simulink library "Banshee_SEL751_Woodward_lib"  (Simulink 8.1)
settings: Solver=ode45  StartTime=0.0  StopTime=10.0  RelTol=1e-3
undefined symbols (not defined in the file): fdesignblkfcn, gcbh
libraries: rtio_opalrt_common x13, simulink x13, rtio_opalrt_op5142ex1 x12, simulink_extras x8, dspswit3 x6
(part 1 of 2)
settings Model: Creator=re25624  LastModifiedBy=re25624

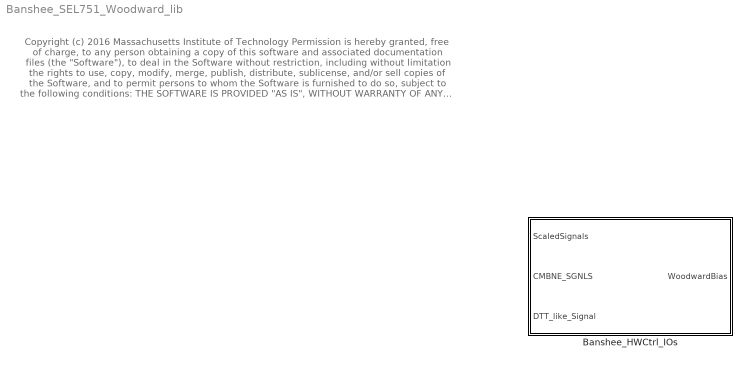
== system Banshee_SEL751_Woodward_lib ==
  note: Copyright (c) 2016 Massachusetts Institute of Technology
      | Permission is hereby granted, free of charge, to any person obtaining a copy of this software and associated documentation files (the "Software"), to deal
      | in the Software without restriction, including without limitation the rights to use, copy, modify, merge, publish, distribute, sublicense, and/or sell copies of the
      | Software, and to permit persons to whom the Software is furnished to do so, subject to the following conditions:
      |
      | THE SOFTWARE IS PROVIDED "AS IS", WITHOUT WARRANTY OF ANY KIND, EXPRESS OR IMPLIED, INCLUDING BUT NOT LIMITED TO THE
      | WARRANTIES OF MERCHANTABILITY, FITNESS FOR A PARTICULAR PURPOSE AND NONINFRINGEMENT. IN NO EVENT SHALL THE AUTHORS
      | OR COPYRIGHT HOLDERS BE LIABLE FOR ANY CLAIM, DAMAGES OR OTHER LIABILITY, WHETHER IN AN ACTION OF CONTRACT, TORT OR
      | OTHERWISE, ARISING FROM, OUT OF OR IN CONNECTION WITH THE SOFTWARE OR THE USE OR OTHER DEALINGS IN THE SOFTWARE
  Banshee_HWCtrl_IOs : Subsystem

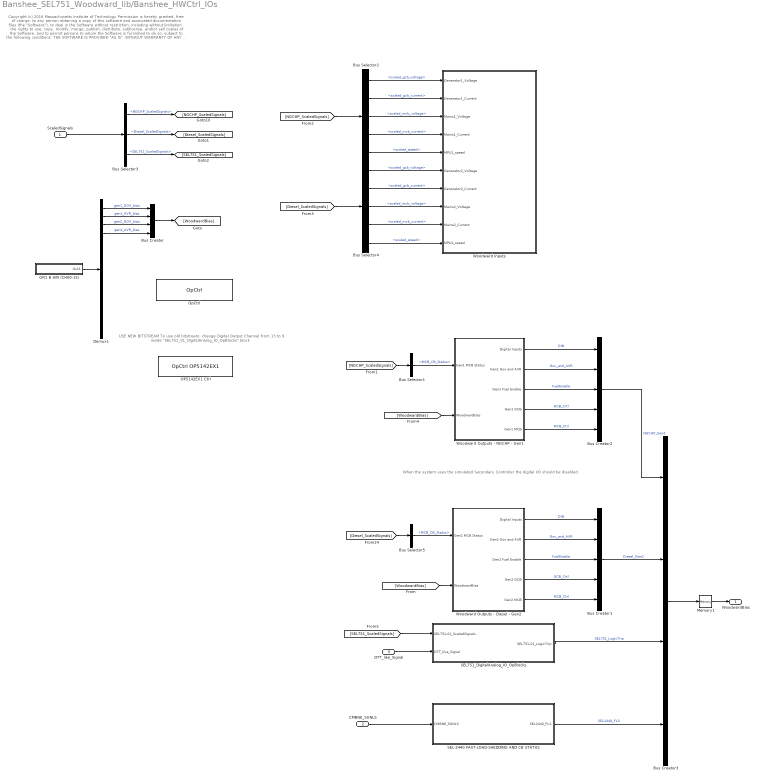
== system Banshee_SEL751_Woodward_lib/Banshee_HWCtrl_IOs ==
  note: USE NEW  BITSTREAM
      | To use old bitstream, change Digital Output Channel from 13 to 9 inside
      | "SEL751_01_DigitalAnalog_IO_OpBlocks" block
  note: Copyright (c) 2016 Massachusetts Institute of Technology
      | Permission is hereby granted, free of charge, to any person obtaining a copy of this software and associated documentation files (the "Software"), to deal
      | in the Software without restriction, including without limitation the rights to use, copy, modify, merge, publish, distribute, sublicense, and/or sell copies of the
      | Software, and to permit persons to whom the Software is furnished to do so, subject to the following conditions:
      |
      | THE SOFTWARE IS PROVIDED "AS IS", WITHOUT WARRANTY OF ANY KIND, EXPRESS OR IMPLIED, INCLUDING BUT NOT LIMITED TO THE
      | WARRANTIES OF MERCHANTABILITY, FITNESS FOR A PARTICULAR PURPOSE AND NONINFRINGEMENT. IN NO EVENT SHALL THE AUTHORS
      | OR COPYRIGHT HOLDERS BE LIABLE FOR ANY CLAIM, DAMAGES OR OTHER LIABILITY, WHETHER IN AN ACTION OF CONTRACT, TORT OR
      | OTHERWISE, ARISING FROM, OUT OF OR IN CONNECTION WITH THE SOFTWARE OR THE USE OR OTHER DEALINGS IN THE SOFTWARE
  note: When the system uses the simulated
      | Secondary Controller the digital I/O
      | should be disabled.
  ScaledSignals : Inport
  CMBNE_SGNLS : Inport  Port=2
  DTT_like_Signal : Inport  Port=3
  Bus Creator : BusCreator
  Bus Creator1 : BusCreator  Inputs=5
  Bus Creator2 : BusCreator  Inputs=5
  Bus Creator3 : BusCreator
  Bus Selector1 : BusSelector  OutputSignals=MCB_CB_Status
  Bus Selector2 : BusSelector  OutputSignals=scaled_gcb_voltage,scaled_gcb_current,scaled_mcb_voltage,scaled_mcb_current,scaled_speed
  Bus Selector3 : BusSelector  OutputSignals=NGCHP_ScaledSignals,Diesel_ScaledSignals,SEL751_ScaledSignals
  Bus Selector4 : BusSelector  OutputSignals=scaled_gcb_voltage,scaled_gcb_current,scaled_mcb_voltage,scaled_mcb_current,scaled_speed
  Bus Selector5 : BusSelector  OutputSignals=MCB_CB_Status
  Demux1 : Demux  Outputs=16
  GR1 B AIN (CH00-15) : Subsystem
  Memory1 : Memory
  OP5142EX1 Ctrl : rtio_opalrt_op5142ex1/OpCtrl OP5142EX1  CtrlName='OP5142EX1 Ctrl'  boardid=1  BitstreamFilename=OP5142_1-EX-0000-2_3_4_54-16AIO_48AO_32DO_16DIO_16selDIO_CD-FF-01.bin  numconfig=-1  mode=Slave  externalClock=off  decimRtsi=0  calibIO=off  SampleTime=0  loadinport=-1
  OpCtrl : rtio_opalrt_common/OpCtrl  CtrlName='OpCtrl'  boardid=0  BitstreamFilename=VC707_2-EX-0001-2_3_2_20-48AIO16DIO16DIOSel-02-01.bin  numconfig=-1  mode=Master  externalClock=off  decimRtsi=0  calibIO=off  SampleTime=0  loadinport=-1  BoardType=VC707  SecondaryPresent=off  sync_type=Audio
  SEL-2440 FAST-LOAD-SHEDDING AND CB STATUS : Subsystem
  SEL751_DigitalAnalog_IO_OpBlocks : Subsystem
  Woodward Inputs : Subsystem
  Woodward Outputs - Diesel - Gen2 : Subsystem
  Woodward Outputs - NGCHP - Gen1 : Subsystem
  WoodwardBias : Outport
  wires:
  DTT_like_Signal/1 -> SEL751_DigitalAnalog_IO_OpBlocks/2(DTT_like_Signal)
  SEL-2440 FAST-LOAD-SHEDDING AND CB STATUS/1(SEL2440_FLS) -> Bus Creator3/4  "SEL2440_FLS"
  CMBNE_SGNLS/1 -> SEL-2440 FAST-LOAD-SHEDDING AND CB STATUS/1(CMBNE_SGNLS)
  [SEL751_ScaledSignals] -> SEL751_DigitalAnalog_IO_OpBlocks/1(SEL751-01_ScaledSignals)
  Bus Selector3/3 -> [SEL751_ScaledSignals]  "<SEL751_ScaledSignals>"
  SEL751_DigitalAnalog_IO_OpBlocks/1(SEL751-01_LogicTrip) -> Bus Creator3/3  "SEL751_LogicTrip"
  ScaledSignals/1 -> Bus Selector3/1
  Bus Selector3/1 -> [NGCHP_ScaledSignals]  "<NGCHP_ScaledSignals>"
  Bus Selector3/2 -> [Diesel_ScaledSignals]  "<Diesel_ScaledSignals>"
  [NGCHP_ScaledSignals] -> Bus Selector2/1
  Bus Selector2/5 -> Woodward Inputs/5(MPU1_speed)  "<scaled_speed>"
  Bus Selector2/4 -> Woodward Inputs/4(Mains1_Current)  "<scaled_mcb_current>"
  Bus Selector2/3 -> Woodward Inputs/3(Mains1_Voltage)  "<scaled_mcb_voltage>"
  Bus Selector2/2 -> Woodward Inputs/2(Generator1_Current)  "<scaled_gcb_current>"
  Bus Selector2/1 -> Woodward Inputs/1(Generator1_Voltage)  "<scaled_gcb_voltage>"
  [Diesel_ScaledSignals] -> Bus Selector4/1
  Bus Selector4/1 -> Woodward Inputs/6(Generator2_Voltage)  "<scaled_gcb_voltage>"
  Bus Selector4/2 -> Woodward Inputs/7(Generator2_Current)  "<scaled_gcb_current>"
  Bus Selector4/3 -> Woodward Inputs/8(Mains2_Voltage)  "<scaled_mcb_voltage>"
  Bus Selector4/4 -> Woodward Inputs/9(Mains2_Current)  "<scaled_mcb_current>"
  Bus Selector4/5 -> Woodward Inputs/10(MPU2_speed)  "<scaled_speed>"
  GR1 B AIN (CH00-15)/1(Out1) -> Demux1/1
  Demux1/1 -> Bus Creator/1  "gen1_GOV_bias"
  Demux1/2 -> Bus Creator/2  "gen1_AVR_bias"
  Demux1/3 -> Bus Creator/3  "gen2_GOV_bias"
  Demux1/4 -> Bus Creator/4  "gen2_AVR_bias"
  Bus Selector5/1 -> Woodward Outputs - Diesel - Gen2/1(Gen2 MCB Status)  "<MCB_CB_Status>"
  [WoodwardBias] -> Woodward Outputs - Diesel - Gen2/2(WoodwardBias)
  [Diesel_ScaledSignals] -> Bus Selector5/1
  Woodward Outputs - Diesel - Gen2/2(Gen2 Gov and AVR) -> Bus Creator1/2  "Gov_and_AVR"
  Woodward Outputs - Diesel - Gen2/3(Gen2 Fuel Enable) -> Bus Creator1/3  "FuelEnable"
  Woodward Outputs - Diesel - Gen2/4(Gen2 GCB) -> Bus Creator1/4  "GCB_Crtl"
  Woodward Outputs - Diesel - Gen2/5(Gen2 MCB) -> Bus Creator1/5  "MCB_Ctrl"
  Bus Creator1/1 -> Bus Creator3/2  "Diesel_Gen2"
  Bus Creator3/1 -> Memory1/1
  Bus Creator2/1 -> Bus Creator3/1  "NGCHP_Gen1"
  Woodward Outputs - NGCHP - Gen1/1(Digital Inputs) -> Bus Creator2/1  "DIN"
  Woodward Outputs - NGCHP - Gen1/2(Gen1 Gov and AVR) -> Bus Creator2/2  "Gov_and_AVR"
  Woodward Outputs - NGCHP - Gen1/3(Gen1 Fuel Enable) -> Bus Creator2/3  "FuelEnable"
  Woodward Outputs - NGCHP - Gen1/4(Gen1 GCB) -> Bus Creator2/4  "GCB_Crtl"
  Woodward Outputs - Diesel - Gen2/1(Digital Inputs) -> Bus Creator1/1  "DIN"
  Woodward Outputs - NGCHP - Gen1/5(Gen1 MCB) -> Bus Creator2/5  "MCB_Ctrl"
  [WoodwardBias] -> Woodward Outputs - NGCHP - Gen1/2(WoodwardBias)
  [NGCHP_ScaledSignals] -> Bus Selector1/1
  Bus Selector1/1 -> Woodward Outputs - NGCHP - Gen1/1(Gen1 MCB Status)  "<MCB_CB_Status>"
  Memory1/1 -> WoodwardBias/1
  Bus Creator/1 -> [WoodwardBias]

== system Banshee_SEL751_Woodward_lib/Banshee_HWCtrl_IOs/GR1 B AIN (CH00-15) ==
  AnalogIn : rtio_opalrt_common/AnalogIn  CtrlName='OpCtrl'  portNb=1  FcnNos=Slot 1 Module B Subsection 1  size=16  maxcount=8  count=8  numchan=8  sampleTime=0
      settings: AttributesFormatString=%<CtrlName>
  AnalogIn1 : rtio_opalrt_common/AnalogIn  CtrlName='OpCtrl'  portNb=2  FcnNos=Slot 1 Module B Subsection 2  size=16  maxcount=8  count=8  numchan=8  sampleTime=0
      settings: AttributesFormatString=%<CtrlName>
  Mux6 : Mux  Inputs=2
  Terminator2 : Terminator
  Terminator3 : Terminator
  Out1 : Outport
  wires:
  AnalogIn/1 -> Mux6/1
  AnalogIn1/1 -> Mux6/2
  AnalogIn/2 -> Terminator2/1
  AnalogIn1/2 -> Terminator3/1
  Mux6/1 -> Out1/1

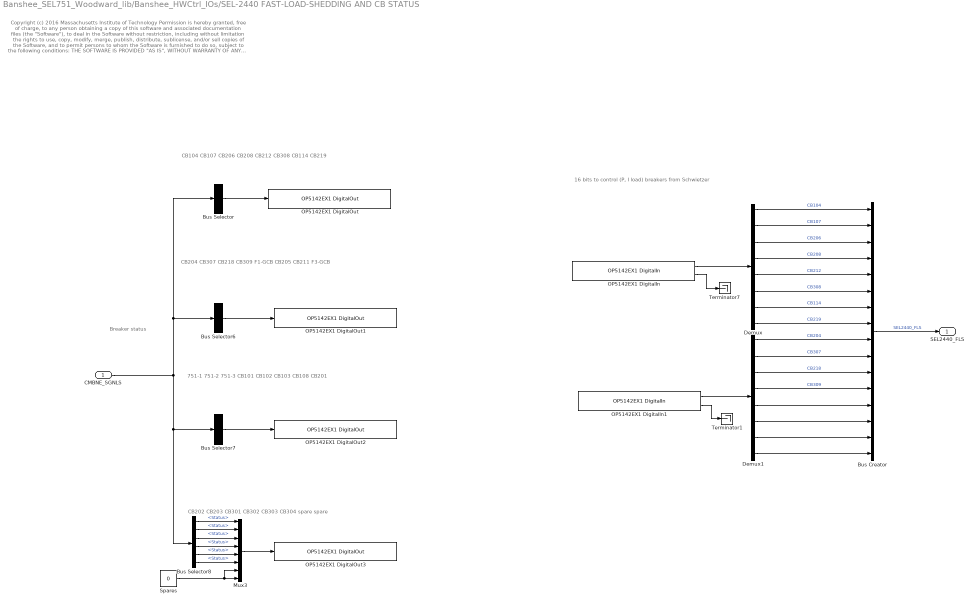
== system Banshee_SEL751_Woodward_lib/Banshee_HWCtrl_IOs/SEL-2440 FAST-LOAD-SHEDDING AND CB STATUS ==
  note: 16 bits to control (P, I load) breakers from Schwietzer
  note: Copyright (c) 2016 Massachusetts Institute of Technology
      | Permission is hereby granted, free of charge, to any person obtaining a copy of this software and associated documentation files (the "Software"), to deal
      | in the Software without restriction, including without limitation the rights to use, copy, modify, merge, publish, distribute, sublicense, and/or sell copies of the
      | Software, and to permit persons to whom the Software is furnished to do so, subject to the following conditions:
      |
      | THE SOFTWARE IS PROVIDED "AS IS", WITHOUT WARRANTY OF ANY KIND, EXPRESS OR IMPLIED, INCLUDING BUT NOT LIMITED TO THE
      | WARRANTIES OF MERCHANTABILITY, FITNESS FOR A PARTICULAR PURPOSE AND NONINFRINGEMENT. IN NO EVENT SHALL THE AUTHORS
      | OR COPYRIGHT HOLDERS BE LIABLE FOR ANY CLAIM, DAMAGES OR OTHER LIABILITY, WHETHER IN AN ACTION OF CONTRACT, TORT OR
      | OTHERWISE, ARISING FROM, OUT OF OR IN CONNECTION WITH THE SOFTWARE OR THE USE OR OTHER DEALINGS IN THE SOFTWARE
  note: CB104
      | CB107
      | CB206
      | CB208
      | CB212
      | CB308
      | CB114
      | CB219
  note: CB204
      | CB307
      | CB218
      | CB309
      | F1-GCB
      | CB205
      | CB211
      | F3-GCB
  note: 751-1
      | 751-2
      | 751-3
      | CB101
      | CB102
      | CB103
      | CB108
      | CB201
  note: CB202
      | CB203
      | CB301
      | CB302
      | CB303
      | CB304
      | spare
      | spare
  note: Breaker status
  CMBNE_SGNLS : Inport
  Bus Creator : BusCreator  Inputs=16
  Bus Selector : BusSelector  OutputSignals=F1_MS_IN.CB_DATA.F1_CB_4.Status,F1_MS_IN.CB_DATA.F1_CB_7.Status,F2_MS_IN.CB_DATA.F2_CB_6.Status,F2_MS_IN.CB_DATA.F2_CB_8.Status,F2_MS_IN.CB_DATA.F2_CB_12.Status,F3_MS_IN.CB_DATA.F3_CB_8.Status,F1_MS_IN.CB_DATA.F1_CB_14.Status,F2_MS_IN.CB_DATA.F2_CB_19.Status  OutputAsBus=on
  Bus Selector6 : BusSelector  OutputSignals=F2_MS_IN.CB_DATA.F2_CB_4.Status,F3_MS_IN.CB_DATA.F3_CB_7.Status,F2_MS_IN.CB_DATA.F2_CB_18.Status,F3_MS_IN.CB_DATA.F3_CB_9.Status,F1_MS_IN.DIESEL_DATA.DIESEL_GCB.cb_ms.Status,F2_MS_IN.CB_DATA.F2_CB_5.Status,F2_MS_IN.CB_DATA.F2_CB_11.Status,F3_MS_IN.NG_CHP_DATA.NG_CHP_GCB.cb_ms.Status  OutputAsBus=on
  Bus Selector7 : BusSelector  OutputSignals=F1_MS_IN.CB_DATA.F1_PCC.Status,F2_MS_IN.CB_DATA.F2_PCC.Status,F3_MS_IN.CB_DATA.F3_PCC.Status,F1_MS_IN.CB_DATA.F1_CB_1.Status,F1_MS_IN.CB_DATA.F1_CB_2.Status,F1_MS_IN.CB_DATA.F1_CB_3.Status,F1_MS_IN.CB_DATA.F1_CB_8.Status,F2_MS_IN.CB_DATA.F2_CB_1.Status  OutputAsBus=on
  Bus Selector8 : BusSelector  OutputSignals=F2_MS_IN.CB_DATA.F2_CB_2.Status,F2_MS_IN.CB_DATA.F2_CB_3.Status,F3_MS_IN.CB_DATA.F3_CB_1.Status,F3_MS_IN.CB_DATA.F3_CB_2.Status,F3_MS_IN.CB_DATA.F3_CB_3.Status,F3_MS_IN.CB_DATA.F3_CB_4.Status
  Demux : Demux  Outputs=8
  Demux1 : Demux  Outputs=8
  Mux3 : Mux  Inputs=8
  OP5142EX1 DigitalIn : rtio_opalrt_op5142ex1/OP5142EX1 DigitalIn  CtrlName='OP5142EX1 Ctrl'  portNb=3  FcnNos=Slot 4 Module A Subsection 1  size=1  maxcount=8  count=8  sampleTime=0  numchan=8
      settings: AttributesFormatString=%<CtrlName>
  OP5142EX1 DigitalIn1 : rtio_opalrt_op5142ex1/OP5142EX1 DigitalIn  CtrlName='OP5142EX1 Ctrl'  portNb=4  FcnNos=Slot 4 Module A Subsection 2  size=1  maxcount=8  count=8  sampleTime=0  numchan=8
      settings: AttributesFormatString=%<CtrlName>
  OP5142EX1 DigitalOut : rtio_opalrt_op5142ex1/OP5142EX1 DigitalOut  CtrlName='OP5142EX1 Ctrl'  portNb=9  FcnNos=Slot 3 Module B Subsection 1  size=1  maxcount=8  count=8  numchan=8
      settings: AttributesFormatString=%<CtrlName>
  OP5142EX1 DigitalOut1 : rtio_opalrt_op5142ex1/OP5142EX1 DigitalOut  CtrlName='OP5142EX1 Ctrl'  portNb=10  FcnNos=Slot 3 Module B Subsection 2  size=1  maxcount=8  count=8  numchan=8
      settings: AttributesFormatString=%<CtrlName>
  OP5142EX1 DigitalOut2 : rtio_opalrt_op5142ex1/OP5142EX1 DigitalOut  CtrlName='OP5142EX1 Ctrl'  portNb=11  FcnNos=Slot 3 Module B Subsection 3  size=1  maxcount=8  count=8  numchan=8
      settings: AttributesFormatString=%<CtrlName>
  OP5142EX1 DigitalOut3 : rtio_opalrt_op5142ex1/OP5142EX1 DigitalOut  CtrlName='OP5142EX1 Ctrl'  portNb=12  FcnNos=Slot 3 Module B Subsection 4  size=1  maxcount=8  count=8  numchan=8
      settings: AttributesFormatString=%<CtrlName>
  Spares : Constant  Value=0
  Terminator1 : Terminator
  Terminator7 : Terminator
  SEL2440_FLS : Outport
  wires:
  Bus Creator/1 -> SEL2440_FLS/1  "SEL2440_FLS"
  Demux1/1 -> Bus Creator/9  "CB204"
  Demux1/2 -> Bus Creator/10  "CB307"
  Demux1/3 -> Bus Creator/11  "CB218"
  Demux1/4 -> Bus Creator/12  "CB309"
  Demux1/5 -> Bus Creator/13
  Demux1/6 -> Bus Creator/14
  Demux1/8 -> Bus Creator/16
  Demux1/7 -> Bus Creator/15
  Demux/8 -> Bus Creator/8  "CB219"
  Demux/7 -> Bus Creator/7  "CB114"
  Demux/6 -> Bus Creator/6  "CB308"
  Demux/5 -> Bus Creator/5  "CB212"
  Demux/4 -> Bus Creator/4  "CB208"
  Demux/3 -> Bus Creator/3  "CB206"
  Demux/2 -> Bus Creator/2  "CB107"
  Demux/1 -> Bus Creator/1  "CB104"
  OP5142EX1 DigitalIn1/1 -> Demux1/1
  OP5142EX1 DigitalIn/1 -> Demux/1
  OP5142EX1 DigitalIn1/2 -> Terminator1/1
  OP5142EX1 DigitalIn/2 -> Terminator7/1
  Mux3/1 -> OP5142EX1 DigitalOut3/1
  Bus Selector6/1 -> OP5142EX1 DigitalOut1/1
  Bus Selector8/6 -> Mux3/6  "<Status>"
  Bus Selector7/1 -> OP5142EX1 DigitalOut2/1
  Bus Selector8/4 -> Mux3/4  "<Status>"
  Spares/1 -> Mux3/8, Mux3/7
  Bus Selector8/5 -> Mux3/5  "<Status>"
  Bus Selector8/2 -> Mux3/2  "<Status>"
  Bus Selector8/3 -> Mux3/3  "<Status>"
  Bus Selector8/1 -> Mux3/1  "<Status>"
  Bus Selector/1 -> OP5142EX1 DigitalOut/1
  CMBNE_SGNLS/1 -> Bus Selector7/1, Bus Selector8/1, Bus Selector6/1, Bus Selector/1

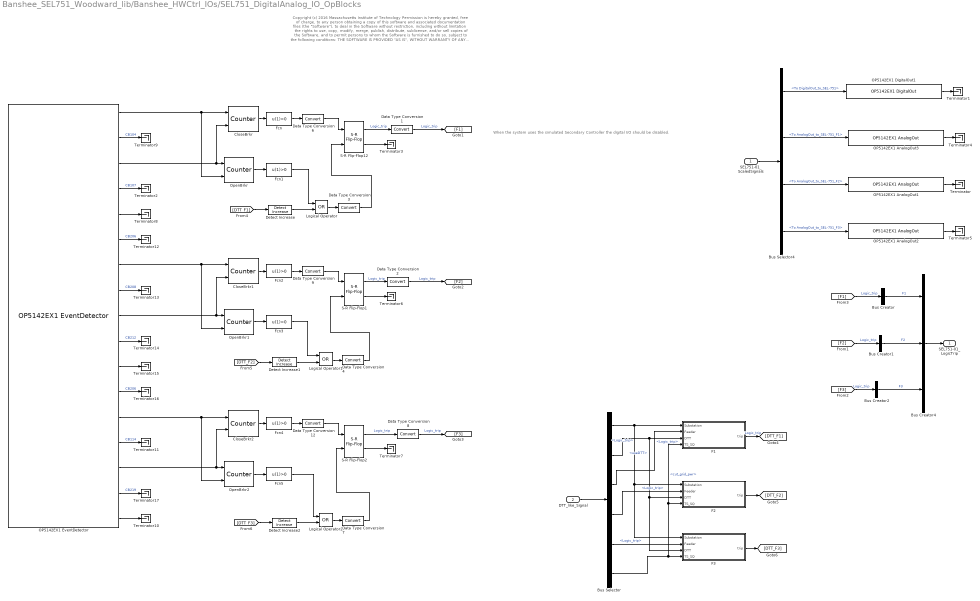
== system Banshee_SEL751_Woodward_lib/Banshee_HWCtrl_IOs/SEL751_DigitalAnalog_IO_OpBlocks ==
  note: Copyright (c) 2016 Massachusetts Institute of Technology
      | Permission is hereby granted, free of charge, to any person obtaining a copy of this software and associated documentation files (the "Software"), to deal
      | in the Software without restriction, including without limitation the rights to use, copy, modify, merge, publish, distribute, sublicense, and/or sell copies of the
      | Software, and to permit persons to whom the Software is furnished to do so, subject to the following conditions:
      |
      | THE SOFTWARE IS PROVIDED "AS IS", WITHOUT WARRANTY OF ANY KIND, EXPRESS OR IMPLIED, INCLUDING BUT NOT LIMITED TO THE
      | WARRANTIES OF MERCHANTABILITY, FITNESS FOR A PARTICULAR PURPOSE AND NONINFRINGEMENT. IN NO EVENT SHALL THE AUTHORS
      | OR COPYRIGHT HOLDERS BE LIABLE FOR ANY CLAIM, DAMAGES OR OTHER LIABILITY, WHETHER IN AN ACTION OF CONTRACT, TORT OR
      | OTHERWISE, ARISING FROM, OUT OF OR IN CONNECTION WITH THE SOFTWARE OR THE USE OR OTHER DEALINGS IN THE SOFTWARE
  note: When the system uses the simulated
      | Secondary Controller the digital I/O
      | should be disabled.
  SEL751-01_ScaledSignals : Inport
  DTT_like_Signal : Inport  Port=2
  Bus Creator : BusCreator  Inputs=1
  Bus Creator1 : BusCreator  Inputs=1
  Bus Creator2 : BusCreator  Inputs=1
  Bus Creator4 : BusCreator  Inputs=3
  Bus Selector : BusSelector  OutputSignals=SC_Signal.GridStatusCtrl.Substation.Logic_trip,SC_Signal.GridStatusCtrl.useDTT,SC_Signal.GridStatusCtrl.Grid_F1.Logic_trip,SC_Signal.GridStatusCtrl.Grid_F2.Logic_trip,SC_Signal.GridStatusCtrl.Grid_F3.Logic_trip,cut_grid_pwr
  Bus Selector4 : BusSelector  OutputSignals=To DigitalOut_to_SEL-751,To AnalogOut_to_SEL-751_F1,To AnalogOut_to_SEL-751_F2,To AnalogOut_to_SEL-751_F3
  CloseBrkr : dspswit3/Counter  Direction=Up  CountEvent=Rising edge  CounterSize=User defined  MaxCount=255  InitialCount=0  Output=Count  HitValue=32  ResetInput=on  SamplesPerFrame=1  Ts=1  CntDtype=double  HitDtype=Logical
  CloseBrkr1 : dspswit3/Counter  Direction=Up  CountEvent=Rising edge  CounterSize=User defined  MaxCount=255  InitialCount=0  Output=Count  HitValue=32  ResetInput=on  SamplesPerFrame=1  Ts=1  CntDtype=double  HitDtype=Logical
  CloseBrkr2 : dspswit3/Counter  Direction=Up  CountEvent=Rising edge  CounterSize=User defined  MaxCount=255  InitialCount=0  Output=Count  HitValue=32  ResetInput=on  SamplesPerFrame=1  Ts=1  CntDtype=double  HitDtype=Logical
  Data Type Conversion{1..4,6..9,12} (9 alike) : DataTypeConversion
  Detect Increase : simulink/Logic and Bit Operations/Detect Increase  vinit=0.0  InputProcessing=Inherited  OutDataTypeStr=boolean
  Detect Increase1 : simulink/Logic and Bit Operations/Detect Increase  vinit=0.0  InputProcessing=Inherited  OutDataTypeStr=boolean
  Detect Increase2 : simulink/Logic and Bit Operations/Detect Increase  vinit=0.0  InputProcessing=Inherited  OutDataTypeStr=boolean
  F1 : Subsystem
  F2 : Subsystem
  F3 : Subsystem
  Fcn{,1..5} (6 alike) : Fcn  Expr=u(1)>0
  Logical Operator : Logic  Operator=OR  AllPortsSameDT=off  OutDataTypeStr=boolean
  Logical Operator1 : Logic  Operator=OR  AllPortsSameDT=off  OutDataTypeStr=boolean
  Logical Operator2 : Logic  Operator=OR  AllPortsSameDT=off  OutDataTypeStr=boolean
  OP5142EX1 AnalogOut1 : rtio_opalrt_op5142ex1/OP5142EX1 AnalogOut  CtrlName='OP5142EX1 Ctrl'  portNb=2  FcnNos=Slot 1 Module A Subsection 2  size=16  maxcount=8  count=8  numchan=8  israngeinput=off  voltagerange=[-16 ... 16]  slot=0  side=0  mismatch=0  slotside=Slot_1_Module_A
      settings: AttributesFormatString=%<CtrlName>
  OP5142EX1 AnalogOut2 : rtio_opalrt_op5142ex1/OP5142EX1 AnalogOut  CtrlName='OP5142EX1 Ctrl'  portNb=3  FcnNos=Slot 2 Module A Subsection 1  size=16  maxcount=8  count=8  numchan=8  israngeinput=off  voltagerange=[-16 ... 16]  slot=1  side=0  mismatch=0  slotside=Slot_2_Module_A
      settings: AttributesFormatString=%<CtrlName>
  OP5142EX1 AnalogOut3 : rtio_opalrt_op5142ex1/OP5142EX1 AnalogOut  CtrlName='OP5142EX1 Ctrl'  portNb=1  FcnNos=Slot 1 Module A Subsection 1  size=16  maxcount=8  count=8  numchan=8  israngeinput=off  voltagerange=[-16 ... 16]  slot=0  side=0  mismatch=0  slotside=Slot_1_Module_A
      settings: AttributesFormatString=%<CtrlName>
  OP5142EX1 DigitalOut1 : rtio_opalrt_op5142ex1/OP5142EX1 DigitalOut  CtrlName='OP5142EX1 Ctrl'  portNb=13  FcnNos=Slot 4 Module B Subsection 1  size=1  maxcount=8  count=8  numchan=8
      settings: AttributesFormatString=%<CtrlName>
  OP5142EX1 EventDetector : rtio_opalrt_op5142ex1/OP5142EX1 EventDetector  CtrlName='OP5142EX1 Ctrl'  portNb=5  FcnNos=Slot 4 Module A Subsection 3  size=32  count=8  nbChannels=8  width=1  timeUnit=Time ratio  sampleTime=0  numwidth=1
      settings: AttributesFormatString=%<CtrlName>
  OpenBrkr : dspswit3/Counter  Direction=Up  CountEvent=Rising edge  CounterSize=User defined  MaxCount=255  InitialCount=0  Output=Count  HitValue=32  ResetInput=on  SamplesPerFrame=1  Ts=1  CntDtype=double  HitDtype=Logical
  OpenBrkr1 : dspswit3/Counter  Direction=Up  CountEvent=Rising edge  CounterSize=User defined  MaxCount=255  InitialCount=0  Output=Count  HitValue=32  ResetInput=on  SamplesPerFrame=1  Ts=1  CntDtype=double  HitDtype=Logical
  OpenBrkr2 : dspswit3/Counter  Direction=Up  CountEvent=Rising edge  CounterSize=User defined  MaxCount=255  InitialCount=0  Output=Count  HitValue=32  ResetInput=on  SamplesPerFrame=1  Ts=1  CntDtype=double  HitDtype=Logical
  S-R Flip-Flop1 : simulink_extras/Flip Flops/S-R Flip-Flop  initial_condition=1
  S-R Flip-Flop12 : simulink_extras/Flip Flops/S-R Flip-Flop  initial_condition=1
  S-R Flip-Flop2 : simulink_extras/Flip Flops/S-R Flip-Flop  initial_condition=1
  Terminator{,1..17} (18 alike) : Terminator
  SEL751-01_LogicTrip : Outport
  wires:
  Bus Selector/6 -> F3/4(TS_SQ), F2/4(TS_SQ), F1/4(TS_SQ)  "<cut_grid_pwr>"
  Data Type Conversion7/1 -> S-R Flip-Flop2/2
  Fcn5/1 -> Logical Operator2/1
  Fcn3/1 -> Logical Operator1/1
  Data Type Conversion4/1 -> S-R Flip-Flop1/2
  Logical Operator2/1 -> Data Type Conversion7/1
  Detect Increase2/1 -> Logical Operator2/2
  [DTT_F3] -> Detect Increase2/1
  Logical Operator1/1 -> Data Type Conversion4/1
  Detect Increase1/1 -> Logical Operator1/2
  [DTT_F2] -> Detect Increase1/1
  Logical Operator/1 -> Data Type Conversion3/1
  Detect Increase/1 -> Logical Operator/2
  [DTT_F1] -> Detect Increase/1
  F3/1(trip) -> [DTT_F3]
  F2/1(trip) -> [DTT_F2]
  F1/1(trip) -> [DTT_F1]  "Logic_trip"
  Bus Selector/5 -> F3/2(Feeder)  "<Logic_trip>"
  Bus Selector/4 -> F2/2(Feeder)  "<Logic_trip>"
  Bus Selector/3 -> F1/2(Feeder)  "<Logic_trip>"
  Bus Selector/2 -> F1/3(DTT), F2/3(DTT), F3/3(DTT)  "<useDTT>"
  Bus Selector/1 -> F1/1(Substation), F3/1(Substation), F2/1(Substation)  "<Logic_trip>"
  [F3] -> Bus Creator2/1  "Logic_trip"
  [F2] -> Bus Creator1/1  "Logic_trip"
  [F1] -> Bus Creator/1  "Logic_trip"
  DTT_like_Signal/1 -> Bus Selector/1
  S-R Flip-Flop2/2 -> Terminator7/1
  S-R Flip-Flop1/2 -> Terminator6/1
  S-R Flip-Flop12/2 -> Terminator3/1
  OP5142EX1 EventDetector/17 -> Terminator10/1
  OP5142EX1 EventDetector/12 -> Terminator16/1  "CB206"
  OP5142EX1 EventDetector/11 -> Terminator15/1
  OP5142EX1 EventDetector/10 -> Terminator14/1  "CB212"
  OP5142EX1 EventDetector/8 -> Terminator13/1  "CB208"
  OP5142EX1 EventDetector/6 -> Terminator12/1  "CB206"
  OP5142EX1 EventDetector/5 -> Terminator8/1
  OP5142EX1 EventDetector/4 -> Terminator2/1  "CB107"
  OP5142EX1 EventDetector/2 -> Terminator9/1  "CB104"
  OP5142EX1 EventDetector/15 -> CloseBrkr2/2, OpenBrkr2/1
  OP5142EX1 EventDetector/13 -> OpenBrkr2/2, CloseBrkr2/1
  Data Type Conversion12/1 -> S-R Flip-Flop2/1
  Fcn4/1 -> Data Type Conversion12/1
  OpenBrkr2/1 -> Fcn5/1
  CloseBrkr2/1 -> Fcn4/1
  OP5142EX1 EventDetector/9 -> CloseBrkr1/2, OpenBrkr1/1
  OP5142EX1 EventDetector/7 -> OpenBrkr1/2, CloseBrkr1/1
  Data Type Conversion9/1 -> S-R Flip-Flop1/1
  Fcn2/1 -> Data Type Conversion9/1
  OpenBrkr1/1 -> Fcn3/1
  CloseBrkr1/1 -> Fcn2/1
  OP5142EX1 EventDetector/3 -> CloseBrkr/2, OpenBrkr/1
  OP5142EX1 EventDetector/1 -> OpenBrkr/2, CloseBrkr/1
  Data Type Conversion3/1 -> S-R Flip-Flop12/2
  Data Type Conversion6/1 -> S-R Flip-Flop12/1
  Fcn1/1 -> Logical Operator/1
  Fcn/1 -> Data Type Conversion6/1
  OpenBrkr/1 -> Fcn1/1
  CloseBrkr/1 -> Fcn/1
  OP5142EX1 EventDetector/16 -> Terminator17/1  "CB219"
  OP5142EX1 EventDetector/14 -> Terminator11/1  "CB114"
  Bus Selector4/2 -> OP5142EX1 AnalogOut3/1  "<To AnalogOut_to_SEL-751_F1>"
  Bus Selector4/3 -> OP5142EX1 AnalogOut1/1  "<To AnalogOut_to_SEL-751_F2>"
  Bus Selector4/4 -> OP5142EX1 AnalogOut2/1  "<To AnalogOut_to_SEL-751_F3>"
  S-R Flip-Flop2/1 -> Data Type Conversion8/1  "Logic_trip"
  S-R Flip-Flop12/1 -> Data Type Conversion1/1  "Logic_trip"
  S-R Flip-Flop1/1 -> Data Type Conversion2/1  "Logic_trip"
  OP5142EX1 AnalogOut3/1 -> Terminator4/1
  OP5142EX1 AnalogOut2/1 -> Terminator5/1
  SEL751-01_ScaledSignals/1 -> Bus Selector4/1
  Bus Selector4/1 -> OP5142EX1 DigitalOut1/1  "<To DigitalOut_to_SEL-751>"
  OP5142EX1 AnalogOut1/1 -> Terminator/1
  OP5142EX1 DigitalOut1/1 -> Terminator1/1
  Bus Creator1/1 -> Bus Creator4/2  "F2"
  Bus Creator2/1 -> Bus Creator4/3  "F3"
  Bus Creator/1 -> Bus Creator4/1  "F1"
  Data Type Conversion8/1 -> [F3]  "Logic_trip"
  Data Type Conversion2/1 -> [F2]  "Logic_trip"
  Bus Creator4/1 -> SEL751-01_LogicTrip/1
  Data Type Conversion1/1 -> [F1]  "Logic_trip"

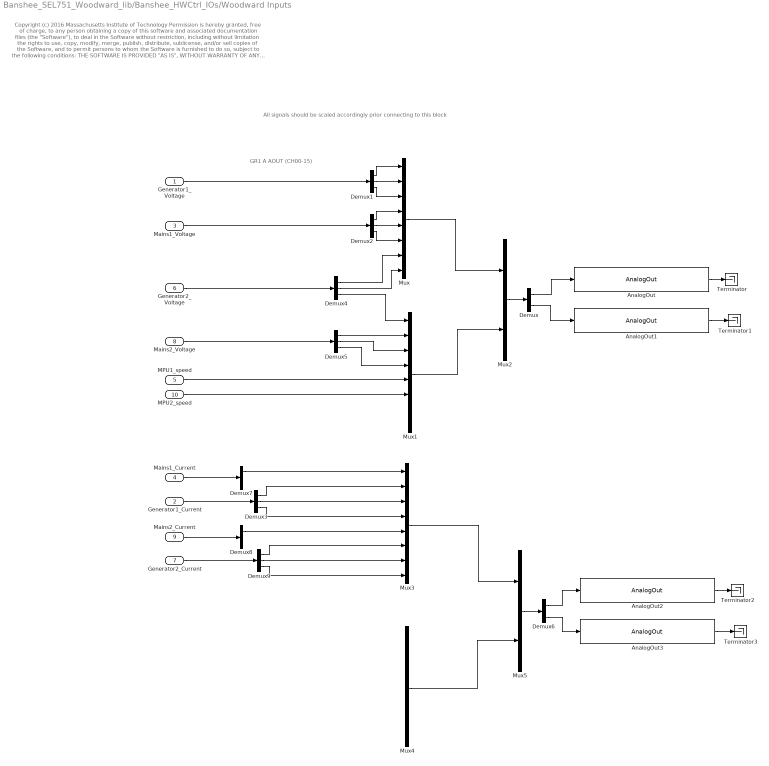
== system Banshee_SEL751_Woodward_lib/Banshee_HWCtrl_IOs/Woodward Inputs ==
  note: All signals should be scaled accordingly prior connecting to this block
  note: GR1 A AOUT (CH00-15)
  note: Copyright (c) 2016 Massachusetts Institute of Technology
      | Permission is hereby granted, free of charge, to any person obtaining a copy of this software and associated documentation files (the "Software"), to deal
      | in the Software without restriction, including without limitation the rights to use, copy, modify, merge, publish, distribute, sublicense, and/or sell copies of the
      | Software, and to permit persons to whom the Software is furnished to do so, subject to the following conditions:
      |
      | THE SOFTWARE IS PROVIDED "AS IS", WITHOUT WARRANTY OF ANY KIND, EXPRESS OR IMPLIED, INCLUDING BUT NOT LIMITED TO THE
      | WARRANTIES OF MERCHANTABILITY, FITNESS FOR A PARTICULAR PURPOSE AND NONINFRINGEMENT. IN NO EVENT SHALL THE AUTHORS
      | OR COPYRIGHT HOLDERS BE LIABLE FOR ANY CLAIM, DAMAGES OR OTHER LIABILITY, WHETHER IN AN ACTION OF CONTRACT, TORT OR
      | OTHERWISE, ARISING FROM, OUT OF OR IN CONNECTION WITH THE SOFTWARE OR THE USE OR OTHER DEALINGS IN THE SOFTWARE
  Generator1_Voltage : Inport
  Generator1_Current : Inport  Port=2
  Mains1_Voltage : Inport  Port=3
  Mains1_Current : Inport  Port=4
  MPU1_speed : Inport  Port=5
  Generator2_Voltage : Inport  Port=6
  Generator2_Current : Inport  Port=7
  Mains2_Voltage : Inport  Port=8
  Mains2_Current : Inport  Port=9
  MPU2_speed : Inport  Port=10
  AnalogOut : rtio_opalrt_common/AnalogOut  CtrlName='OpCtrl'  portNb=1  FcnNos=Slot 1 Module A Subsection 1  size=16  maxcount=8  count=8  numchan=8  israngeinput=off  voltagerange=[-16 ... 16]  slot=0  side=0  mismatch=0  slotside=Slot_1_Module_A
      settings: AttributesFormatString=%<CtrlName>
  AnalogOut1 : rtio_opalrt_common/AnalogOut  CtrlName='OpCtrl'  portNb=2  FcnNos=Slot 1 Module A Subsection 2  size=16  maxcount=8  count=8  numchan=8  israngeinput=off  voltagerange=[-16 ... 16]  slot=0  side=0  mismatch=0  slotside=Slot_1_Module_A
      settings: AttributesFormatString=%<CtrlName>
  AnalogOut2 : rtio_opalrt_common/AnalogOut  CtrlName='OpCtrl'  portNb=3  FcnNos=Slot 2 Module A Subsection 1  size=16  maxcount=8  count=8  numchan=8  israngeinput=off  voltagerange=[-16 ... 16]  slot=1  side=0  mismatch=0  slotside=Slot_2_Module_A
      settings: AttributesFormatString=%<CtrlName>
  AnalogOut3 : rtio_opalrt_common/AnalogOut  CtrlName='OpCtrl'  portNb=4  FcnNos=Slot 2 Module A Subsection 2  size=16  maxcount=8  count=8  numchan=8  israngeinput=off  voltagerange=[-16 ... 16]  slot=1  side=0  mismatch=0  slotside=Slot_2_Module_A
      settings: AttributesFormatString=%<CtrlName>
  Demux : Demux  Outputs=2
  Demux{1..5,7..9} (8 alike) : Demux  Outputs=3
  Demux6 : Demux  Outputs=2
  Mux{,1,3..4} (4 alike) : Mux  Inputs=8
  Mux2 : Mux  Inputs=2
  Mux5 : Mux  Inputs=2
  Terminator{,1..3} (4 alike) : Terminator
  wires:
  Demux9/3 -> Mux3/8
  Demux9/2 -> Mux3/7
  Demux9/1 -> Mux3/6
  Generator2_Current/1 -> Demux9/1
  Demux8/1 -> Mux3/5
  Mains2_Current/1 -> Demux8/1
  MPU2_speed/1 -> Mux1/6
  Generator2_Voltage/1 -> Demux4/1
  Mains2_Voltage/1 -> Demux5/1
  Demux7/1 -> Mux3/1
  Mains1_Current/1 -> Demux7/1
  Demux3/3 -> Mux3/4
  Demux3/2 -> Mux3/3
  Demux3/1 -> Mux3/2
  Generator1_Current/1 -> Demux3/1
  AnalogOut2/1 -> Terminator2/1
  AnalogOut3/1 -> Terminator3/1
  Demux6/1 -> AnalogOut2/1
  Demux6/2 -> AnalogOut3/1
  Mux3/1 -> Mux5/1
  Mux4/1 -> Mux5/2
  Mux5/1 -> Demux6/1
  Demux5/3 -> Mux1/4
  Demux5/2 -> Mux1/3
  Demux5/1 -> Mux1/2
  Demux4/3 -> Mux1/1
  Demux4/2 -> Mux/8
  Demux4/1 -> Mux/7
  MPU1_speed/1 -> Mux1/5
  Demux2/3 -> Mux/6
  Demux2/2 -> Mux/5
  Demux2/1 -> Mux/4
  Demux1/3 -> Mux/3
  Demux1/2 -> Mux/2
  Demux1/1 -> Mux/1
  AnalogOut/1 -> Terminator/1
  AnalogOut1/1 -> Terminator1/1
  Demux/1 -> AnalogOut/1
  Demux/2 -> AnalogOut1/1
  Mux/1 -> Mux2/1
  Mux1/1 -> Mux2/2
  Mux2/1 -> Demux/1
  Generator1_Voltage/1 -> Demux1/1
  Mains1_Voltage/1 -> Demux2/1

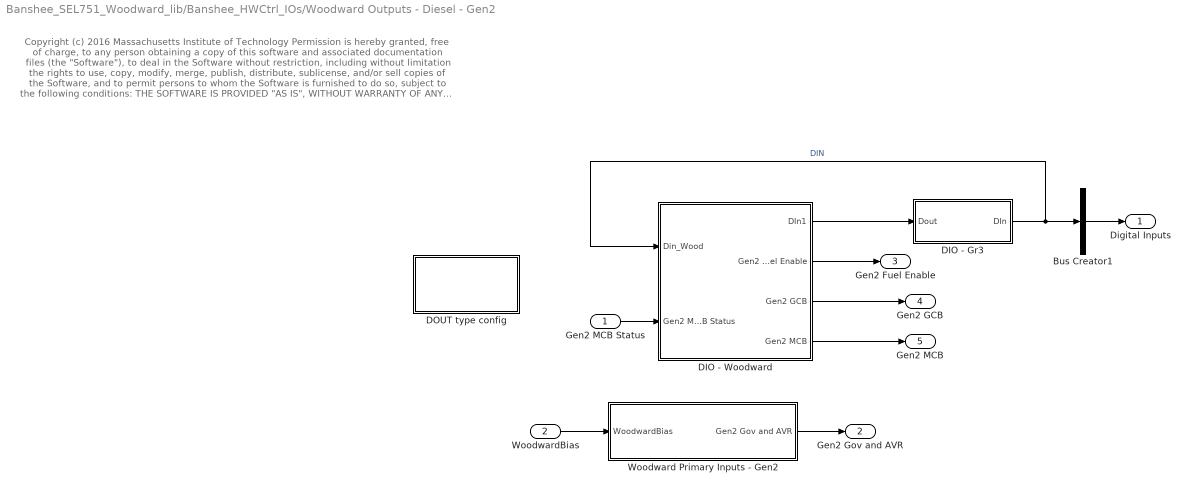
== system Banshee_SEL751_Woodward_lib/Banshee_HWCtrl_IOs/Woodward Outputs - Diesel - Gen2 ==
  note: Copyright (c) 2016 Massachusetts Institute of Technology
      | Permission is hereby granted, free of charge, to any person obtaining a copy of this software and associated documentation files (the "Software"), to deal
      | in the Software without restriction, including without limitation the rights to use, copy, modify, merge, publish, distribute, sublicense, and/or sell copies of the
      | Software, and to permit persons to whom the Software is furnished to do so, subject to the following conditions:
      |
      | THE SOFTWARE IS PROVIDED "AS IS", WITHOUT WARRANTY OF ANY KIND, EXPRESS OR IMPLIED, INCLUDING BUT NOT LIMITED TO THE
      | WARRANTIES OF MERCHANTABILITY, FITNESS FOR A PARTICULAR PURPOSE AND NONINFRINGEMENT. IN NO EVENT SHALL THE AUTHORS
      | OR COPYRIGHT HOLDERS BE LIABLE FOR ANY CLAIM, DAMAGES OR OTHER LIABILITY, WHETHER IN AN ACTION OF CONTRACT, TORT OR
      | OTHERWISE, ARISING FROM, OUT OF OR IN CONNECTION WITH THE SOFTWARE OR THE USE OR OTHER DEALINGS IN THE SOFTWARE
  Gen2 MCB Status : Inport
  WoodwardBias : Inport  Port=2
  Bus Creator1 : BusCreator  Inputs=1
  DIO - Gr3 : Subsystem
  DIO - Woodward : Subsystem
  DOUT type config : Subsystem
  Woodward Primary Inputs - Gen2 : Subsystem
  Digital Inputs : Outport
  Gen2 Gov and AVR : Outport  Port=2
  Gen2 Fuel Enable : Outport  Port=3
  Gen2 GCB : Outport  Port=4
  Gen2 MCB : Outport  Port=5
  wires:
  WoodwardBias/1 -> Woodward Primary Inputs - Gen2/1(WoodwardBias)
  Gen2 MCB Status/1 -> DIO - Woodward/2(Gen2 MCB Status)
  DIO - Woodward/4(Gen2 MCB) -> Gen2 MCB/1
  DIO - Woodward/2(Gen2 Fuel Enable) -> Gen2 Fuel Enable/1
  DIO - Woodward/3(Gen2 GCB) -> Gen2 GCB/1
  Woodward Primary Inputs - Gen2/1(Gen2 Gov and AVR) -> Gen2 Gov and AVR/1
  DIO - Gr3/1(DIn) -> DIO - Woodward/1(Din_Wood), Bus Creator1/1  "DIN"
  DIO - Woodward/1(DIn1) -> DIO - Gr3/1(Dout)
  Bus Creator1/1 -> Digital Inputs/1

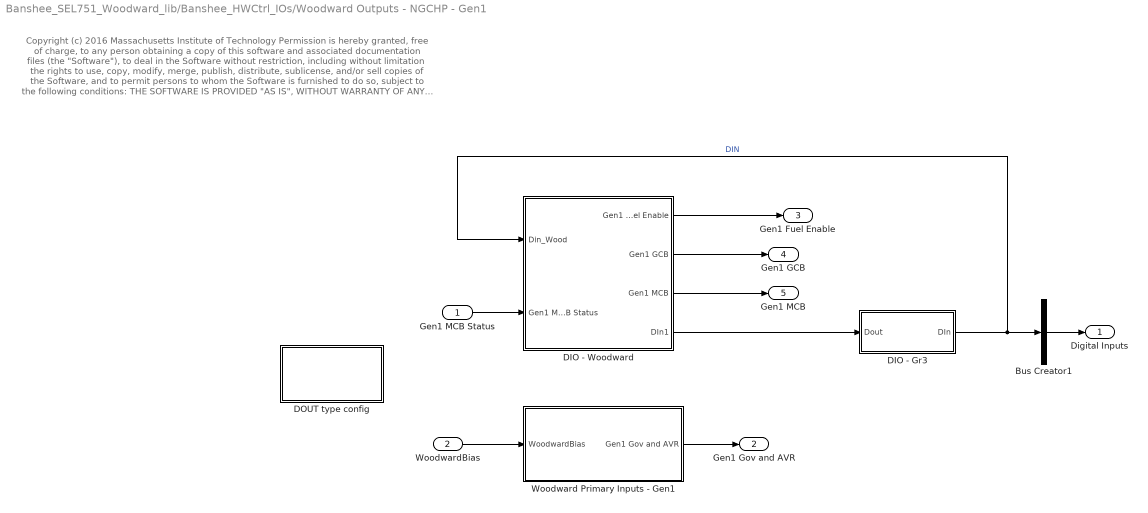
== system Banshee_SEL751_Woodward_lib/Banshee_HWCtrl_IOs/Woodward Outputs - NGCHP - Gen1 ==
  note: Copyright (c) 2016 Massachusetts Institute of Technology
      | Permission is hereby granted, free of charge, to any person obtaining a copy of this software and associated documentation files (the "Software"), to deal
      | in the Software without restriction, including without limitation the rights to use, copy, modify, merge, publish, distribute, sublicense, and/or sell copies of the
      | Software, and to permit persons to whom the Software is furnished to do so, subject to the following conditions:
      |
      | THE SOFTWARE IS PROVIDED "AS IS", WITHOUT WARRANTY OF ANY KIND, EXPRESS OR IMPLIED, INCLUDING BUT NOT LIMITED TO THE
      | WARRANTIES OF MERCHANTABILITY, FITNESS FOR A PARTICULAR PURPOSE AND NONINFRINGEMENT. IN NO EVENT SHALL THE AUTHORS
      | OR COPYRIGHT HOLDERS BE LIABLE FOR ANY CLAIM, DAMAGES OR OTHER LIABILITY, WHETHER IN AN ACTION OF CONTRACT, TORT OR
      | OTHERWISE, ARISING FROM, OUT OF OR IN CONNECTION WITH THE SOFTWARE OR THE USE OR OTHER DEALINGS IN THE SOFTWARE
  Gen1 MCB Status : Inport
  WoodwardBias : Inport  Port=2
  Bus Creator1 : BusCreator  Inputs=1
  DIO - Gr3 : Subsystem
  DIO - Woodward : Subsystem
  DOUT type config : Subsystem
  Woodward Primary Inputs - Gen1 : Subsystem
  Digital Inputs : Outport
  Gen1 Gov and AVR : Outport  Port=2
  Gen1 Fuel Enable : Outport  Port=3
  Gen1 GCB : Outport  Port=4
  Gen1 MCB : Outport  Port=5
  wires:
  Gen1 MCB Status/1 -> DIO - Woodward/2(Gen1 MCB Status)
  DIO - Woodward/1(Gen1 Fuel Enable) -> Gen1 Fuel Enable/1
  DIO - Woodward/3(Gen1 MCB) -> Gen1 MCB/1
  DIO - Woodward/2(Gen1 GCB) -> Gen1 GCB/1
  WoodwardBias/1 -> Woodward Primary Inputs - Gen1/1(WoodwardBias)
  Woodward Primary Inputs - Gen1/1(Gen1 Gov and AVR) -> Gen1 Gov and AVR/1
  Bus Creator1/1 -> Digital Inputs/1
  DIO - Gr3/1(DIn) -> Bus Creator1/1, DIO - Woodward/1(Din_Wood)  "DIN"
  DIO - Woodward/4(DIn1) -> DIO - Gr3/1(Dout)

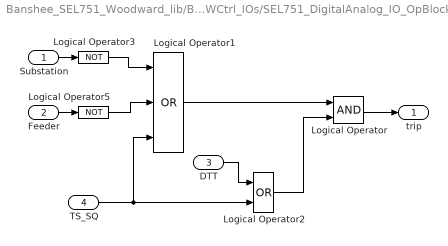
== system Banshee_SEL751_Woodward_lib/Banshee_HWCtrl_IOs/SEL751_DigitalAnalog_IO_OpBlocks/F1 ==
  Substation : Inport
  Feeder : Inport  Port=2
  DTT : Inport  Port=3
  TS_SQ : Inport  Port=4
  Logical Operator : Logic  AllPortsSameDT=off  OutDataTypeStr=boolean
  Logical Operator1 : Logic  Operator=OR  Inputs=3  AllPortsSameDT=off  OutDataTypeStr=boolean
  Logical Operator2 : Logic  Operator=OR  AllPortsSameDT=off  OutDataTypeStr=boolean
  Logical Operator3 : Logic  Operator=NOT  AllPortsSameDT=off  OutDataTypeStr=boolean
  Logical Operator5 : Logic  Operator=NOT  AllPortsSameDT=off  OutDataTypeStr=boolean
  trip : Outport
  wires:
  TS_SQ/1 -> Logical Operator2/2, Logical Operator1/3
  Logical Operator2/1 -> Logical Operator/2
  Logical Operator/1 -> trip/1
  Logical Operator1/1 -> Logical Operator/1
  Logical Operator3/1 -> Logical Operator1/1
  Substation/1 -> Logical Operator3/1
  Logical Operator5/1 -> Logical Operator1/2
  Feeder/1 -> Logical Operator5/1
  DTT/1 -> Logical Operator2/1

== system Banshee_SEL751_Woodward_lib/Banshee_HWCtrl_IOs/SEL751_DigitalAnalog_IO_OpBlocks/F2 ==
  Substation : Inport
  Feeder : Inport  Port=2
  DTT : Inport  Port=3
  TS_SQ : Inport  Port=4
  Logical Operator : Logic  AllPortsSameDT=off  OutDataTypeStr=boolean
  Logical Operator1 : Logic  Operator=OR  Inputs=3  AllPortsSameDT=off  OutDataTypeStr=boolean
  Logical Operator2 : Logic  Operator=OR  AllPortsSameDT=off  OutDataTypeStr=boolean
  Logical Operator3 : Logic  Operator=NOT  AllPortsSameDT=off  OutDataTypeStr=boolean
  Logical Operator5 : Logic  Operator=NOT  AllPortsSameDT=off  OutDataTypeStr=boolean
  trip : Outport
  wires:
  TS_SQ/1 -> Logical Operator2/2, Logical Operator1/3
  Logical Operator2/1 -> Logical Operator/2
  Logical Operator/1 -> trip/1
  Logical Operator1/1 -> Logical Operator/1
  Logical Operator3/1 -> Logical Operator1/1
  Substation/1 -> Logical Operator3/1
  Logical Operator5/1 -> Logical Operator1/2
  Feeder/1 -> Logical Operator5/1
  DTT/1 -> Logical Operator2/1

== system Banshee_SEL751_Woodward_lib/Banshee_HWCtrl_IOs/SEL751_DigitalAnalog_IO_OpBlocks/F3 ==
  Substation : Inport
  Feeder : Inport  Port=2
  DTT : Inport  Port=3
  TS_SQ : Inport  Port=4
  Logical Operator : Logic  AllPortsSameDT=off  OutDataTypeStr=boolean
  Logical Operator1 : Logic  Operator=OR  Inputs=3  AllPortsSameDT=off  OutDataTypeStr=boolean
  Logical Operator2 : Logic  Operator=OR  AllPortsSameDT=off  OutDataTypeStr=boolean
  Logical Operator3 : Logic  Operator=NOT  AllPortsSameDT=off  OutDataTypeStr=boolean
  Logical Operator5 : Logic  Operator=NOT  AllPortsSameDT=off  OutDataTypeStr=boolean
  trip : Outport
  wires:
  TS_SQ/1 -> Logical Operator2/2, Logical Operator1/3
  Logical Operator2/1 -> Logical Operator/2
  Logical Operator/1 -> trip/1
  Logical Operator1/1 -> Logical Operator/1
  Logical Operator3/1 -> Logical Operator1/1
  Substation/1 -> Logical Operator3/1
  Logical Operator5/1 -> Logical Operator1/2
  Feeder/1 -> Logical Operator5/1
  DTT/1 -> Logical Operator2/1

== system Banshee_SEL751_Woodward_lib/Banshee_HWCtrl_IOs/Woodward Outputs - Diesel - Gen2/DIO - Gr3 ==
  Dout : Inport
  Bus Creator : BusCreator  Inputs=1
  Bus Selector1 : BusSelector  OutputSignals=DI_CH08-15  OutputAsBus=on
  Conditioning1 : Subsystem
  DigitalIn1 : rtio_opalrt_common/DigitalIn  CtrlName='OpCtrl'  portNb=6  FcnNos=Slot 3 Module A Subsection 2  size=1  maxcount=8  count=8  sampleTime=0  numchan=8
      settings: AttributesFormatString=%<CtrlName>
  DigitalOut1 : rtio_opalrt_common/DigitalOut  CtrlName='OpCtrl'  portNb=6  FcnNos=Slot 3 Module B Subsection 2  size=1  maxcount=8  count=8  numchan=8
      settings: AttributesFormatString=%<CtrlName>
  Terminator1 : Terminator
  Terminator6 : Terminator
  DIn : Outport
  wires:
  Conditioning1/1(Out1) -> Bus Creator/1
  Bus Creator/1 -> DIn/1
  DigitalIn1/1 -> Conditioning1/1(In1)  "DI_CH08-15"
  DigitalIn1/2 -> Terminator6/1
  Bus Selector1/1 -> DigitalOut1/1
  Dout/1 -> Bus Selector1/1
  DigitalOut1/1 -> Terminator1/1

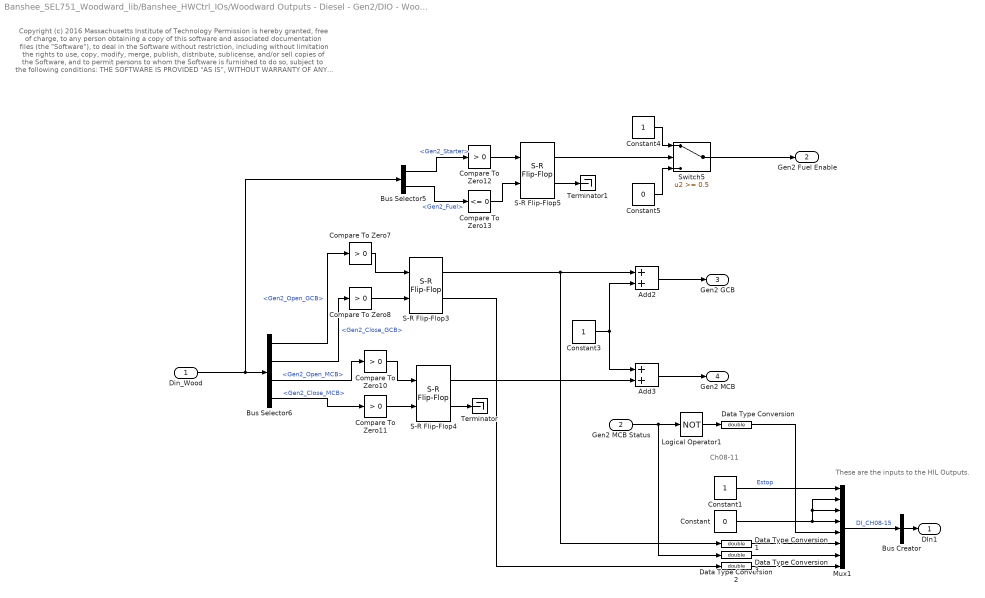
== system Banshee_SEL751_Woodward_lib/Banshee_HWCtrl_IOs/Woodward Outputs - Diesel - Gen2/DIO - Woodward ==
  note: These are the inputs to
      | the HIL Outputs.
  note: Ch08-11
  note: Copyright (c) 2016 Massachusetts Institute of Technology
      | Permission is hereby granted, free of charge, to any person obtaining a copy of this software and associated documentation files (the "Software"), to deal
      | in the Software without restriction, including without limitation the rights to use, copy, modify, merge, publish, distribute, sublicense, and/or sell copies of the
      | Software, and to permit persons to whom the Software is furnished to do so, subject to the following conditions:
      |
      | THE SOFTWARE IS PROVIDED "AS IS", WITHOUT WARRANTY OF ANY KIND, EXPRESS OR IMPLIED, INCLUDING BUT NOT LIMITED TO THE
      | WARRANTIES OF MERCHANTABILITY, FITNESS FOR A PARTICULAR PURPOSE AND NONINFRINGEMENT. IN NO EVENT SHALL THE AUTHORS
      | OR COPYRIGHT HOLDERS BE LIABLE FOR ANY CLAIM, DAMAGES OR OTHER LIABILITY, WHETHER IN AN ACTION OF CONTRACT, TORT OR
      | OTHERWISE, ARISING FROM, OUT OF OR IN CONNECTION WITH THE SOFTWARE OR THE USE OR OTHER DEALINGS IN THE SOFTWARE
  Din_Wood : Inport
  Gen2 MCB Status : Inport  Port=2
  Add2 : Sum
  Add3 : Sum
  Bus Creator : BusCreator  Inputs=1
  Bus Selector5 : BusSelector  OutputSignals=DI_CH08-15.Gen2_Starter,DI_CH08-15.Gen2_Fuel
  Bus Selector6 : BusSelector  OutputSignals=DI_CH08-15.Gen2_Open_GCB,DI_CH08-15.Gen2_Close_GCB,DI_CH08-15.Gen2_Open_MCB,DI_CH08-15.Gen2_Close_MCB
  Compare To Zero{7..8,10..12} (5 alike) : simulink/Logic and Bit Operations/Compare To Zero  relop=>  OutDataTypeStr=boolean
  Compare To Zero13 : simulink/Logic and Bit Operations/Compare To Zero  relop=<=  OutDataTypeStr=boolean
  Constant : Constant  Value=0
  Constant1 : Constant
  Constant3 : Constant
  Constant4 : Constant
  Constant5 : Constant  Value=0
  Data Type Conversion{,1..3} (4 alike) : DataTypeConversion  OutDataTypeStr=double
  Logical Operator1 : Logic  Operator=NOT  AllPortsSameDT=off  OutDataTypeStr=boolean
  Mux1 : Mux  Inputs=8
  S-R Flip-Flop3 : simulink_extras/Flip Flops/S-R Flip-Flop  initial_condition=1
  S-R Flip-Flop4 : simulink_extras/Flip Flops/S-R Flip-Flop  initial_condition=1
  S-R Flip-Flop5 : simulink_extras/Flip Flops/S-R Flip-Flop  initial_condition=0
  Switch5 : Switch  Threshold=0.5
  Terminator : Terminator
  Terminator1 : Terminator
  DIn1 : Outport
  Gen2 Fuel Enable : Outport  Port=2
  Gen2 GCB : Outport  Port=3
  Gen2 MCB : Outport  Port=4
  wires:
  Data Type Conversion/1 -> Mux1/5
  Logical Operator1/1 -> Data Type Conversion/1
  S-R Flip-Flop3/2 -> Data Type Conversion3/1
  Gen2 MCB Status/1 -> Data Type Conversion2/1, Logical Operator1/1
  Switch5/1 -> Gen2 Fuel Enable/1
  Compare To Zero13/1 -> S-R Flip-Flop5/2
  Constant4/1 -> Switch5/1
  Constant5/1 -> Switch5/3
  Compare To Zero12/1 -> S-R Flip-Flop5/1
  S-R Flip-Flop5/1 -> Switch5/2
  Bus Selector5/2 -> Compare To Zero13/1  "<Gen2_Fuel>"
  Bus Selector5/1 -> Compare To Zero12/1  "<Gen2_Starter>"
  Constant3/1 -> Add3/1, Add2/2
  Add3/1 -> Gen2 MCB/1
  Add2/1 -> Gen2 GCB/1
  S-R Flip-Flop4/1 -> Add3/2
  Bus Selector6/2 -> Compare To Zero8/1  "<Gen2_Close_GCB>"
  Compare To Zero10/1 -> S-R Flip-Flop4/1
  Bus Selector6/3 -> Compare To Zero10/1  "<Gen2_Open_MCB>"
  Compare To Zero11/1 -> S-R Flip-Flop4/2
  Bus Selector6/4 -> Compare To Zero11/1  "<Gen2_Close_MCB>"
  Compare To Zero8/1 -> S-R Flip-Flop3/2
  Compare To Zero7/1 -> S-R Flip-Flop3/1
  Bus Selector6/1 -> Compare To Zero7/1  "<Gen2_Open_GCB>"
  S-R Flip-Flop3/1 -> Add2/1, Data Type Conversion1/1
  Mux1/1 -> Bus Creator/1  "DI_CH08-15"
  Bus Creator/1 -> DIn1/1
  Din_Wood/1 -> Bus Selector6/1, Bus Selector5/1
  S-R Flip-Flop4/2 -> Terminator/1
  S-R Flip-Flop5/2 -> Terminator1/1
  Constant/1 -> Mux1/2, Mux1/3, Mux1/4
  Data Type Conversion1/1 -> Mux1/6
  Data Type Conversion2/1 -> Mux1/7
  Data Type Conversion3/1 -> Mux1/8
  Constant1/1 -> Mux1/1  "Estop"

== system Banshee_SEL751_Woodward_lib/Banshee_HWCtrl_IOs/Woodward Outputs - Diesel - Gen2/DOUT type config ==
  note: The Constants are used to select Digital Output type:
      | - 0: Time-Stamped Digital Output
      | - 1: Pulse-Width Modulated DIgital Output
  DataIn Send1 : rtio_opalrt_common/DataIn Send  CtrlName='OpCtrl'  FcnNos=12  width=1  portType=double  checkVersion=off  expectedId=0  expectedVersion=0  opComp=>=
      settings: AttributesFormatString=%<CtrlName>
  Subsection 4 DOUT type : Constant
  Terminator1 : Terminator
  wires:
  DataIn Send1/1 -> Terminator1/1
  Subsection 4 DOUT type/1 -> DataIn Send1/1

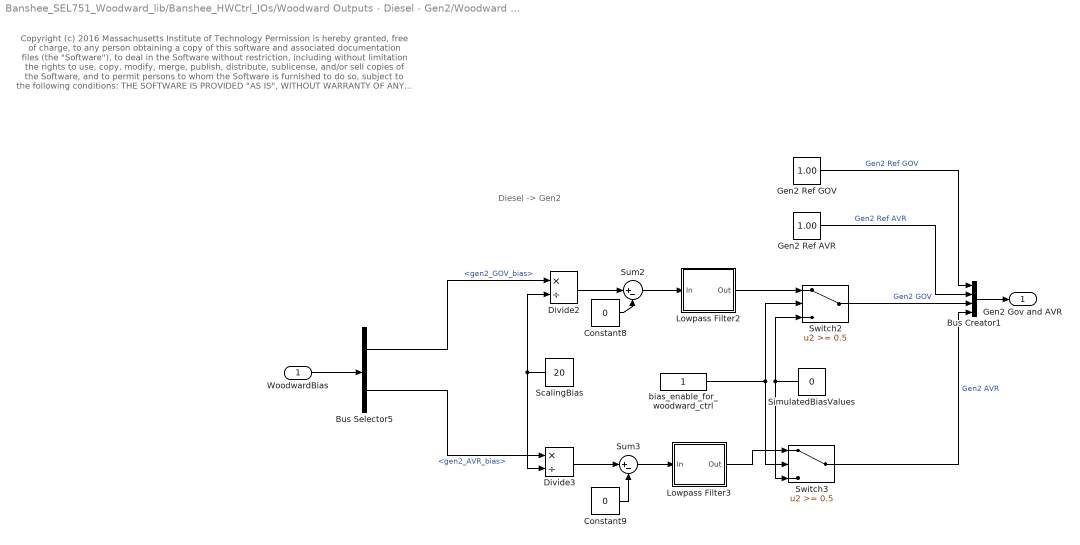
== system Banshee_SEL751_Woodward_lib/Banshee_HWCtrl_IOs/Woodward Outputs - Diesel - Gen2/Woodward Primary Inputs - Gen2 ==
  note: Diesel -> Gen2
  note: Copyright (c) 2016 Massachusetts Institute of Technology
      | Permission is hereby granted, free of charge, to any person obtaining a copy of this software and associated documentation files (the "Software"), to deal
      | in the Software without restriction, including without limitation the rights to use, copy, modify, merge, publish, distribute, sublicense, and/or sell copies of the
      | Software, and to permit persons to whom the Software is furnished to do so, subject to the following conditions:
      |
      | THE SOFTWARE IS PROVIDED "AS IS", WITHOUT WARRANTY OF ANY KIND, EXPRESS OR IMPLIED, INCLUDING BUT NOT LIMITED TO THE
      | WARRANTIES OF MERCHANTABILITY, FITNESS FOR A PARTICULAR PURPOSE AND NONINFRINGEMENT. IN NO EVENT SHALL THE AUTHORS
      | OR COPYRIGHT HOLDERS BE LIABLE FOR ANY CLAIM, DAMAGES OR OTHER LIABILITY, WHETHER IN AN ACTION OF CONTRACT, TORT OR
      | OTHERWISE, ARISING FROM, OUT OF OR IN CONNECTION WITH THE SOFTWARE OR THE USE OR OTHER DEALINGS IN THE SOFTWARE
  WoodwardBias : Inport
  Bus Creator1 : BusCreator
  Bus Selector5 : BusSelector  OutputSignals=gen2_GOV_bias,gen2_AVR_bias
  Constant8 : Constant  Value=0
  Constant9 : Constant  Value=0
  Divide2 : Product  Inputs=*/
  Divide3 : Product  Inputs=*/
  Gen2 Ref AVR : Constant  Value=1.00
  Gen2 Ref GOV : Constant  Value=1.00
  Lowpass Filter2 : Subsystem  DialogController=fdesignblkfcn  DialogControllerArgs=DataTag1  InitFcn=fdesignblkfcn(gcbh, {'InitFcn'});  mask(Lowpass Filter){}
      mask help: Design a lowpass filter
      settings: CopyFcn=fdesignblkfcn(gcbh, {'CopyFcn'});
      mask Help: helpview(mapfilelocation('dsp'), 'dsplowpassfilter');
      mask Display: disp('Lowpass')
  Lowpass Filter3 : Subsystem  DialogController=fdesignblkfcn  DialogControllerArgs=DataTag3  InitFcn=fdesignblkfcn(gcbh, {'InitFcn'});  mask(Lowpass Filter){}
      mask help: Design a lowpass filter
      settings: CopyFcn=fdesignblkfcn(gcbh, {'CopyFcn'});
      mask Help: helpview(mapfilelocation('dsp'), 'dsplowpassfilter');
      mask Display: disp('Lowpass')
  ScalingBias : Constant  Value=20
  SimulatedBiasValues : Constant  Value=0
  Sum2 : Sum  Inputs=|+-
  Sum3 : Sum  Inputs=|+-
  Switch2 : Switch  Threshold=0.5
  Switch3 : Switch  Threshold=0.5
  bias_enable_for_woodward_ctrl : Constant
  Gen2 Gov and AVR : Outport
  wires:
  Bus Selector5/2 -> Divide3/1  "<gen2_AVR_bias>"
  Bus Selector5/1 -> Divide2/1  "<gen2_GOV_bias>"
  WoodwardBias/1 -> Bus Selector5/1
  Bus Creator1/1 -> Gen2 Gov and AVR/1
  Gen2 Ref GOV/1 -> Bus Creator1/1  "Gen2 Ref GOV"
  Gen2 Ref AVR/1 -> Bus Creator1/2  "Gen2 Ref AVR"
  Lowpass Filter3/1(Out) -> Switch3/1
  Lowpass Filter2/1(Out) -> Switch2/1
  SimulatedBiasValues/1 -> Switch3/3, Switch2/3
  Sum3/1 -> Lowpass Filter3/1(In)
  Switch3/1 -> Bus Creator1/4  "Gen2 AVR"
  Switch2/1 -> Bus Creator1/3  "Gen2 GOV"
  Sum2/1 -> Lowpass Filter2/1(In)
  Constant9/1 -> Sum3/2
  Constant8/1 -> Sum2/2
  Divide3/1 -> Sum3/1
  Divide2/1 -> Sum2/1
  ScalingBias/1 -> Divide3/2, Divide2/2
  bias_enable_for_woodward_ctrl/1 -> Switch3/2, Switch2/2

== system Banshee_SEL751_Woodward_lib/Banshee_HWCtrl_IOs/Woodward Outputs - NGCHP - Gen1/DIO - Gr3 ==
  Dout : Inport
  Bus Creator : BusCreator  Inputs=1
  Bus Selector : BusSelector  OutputSignals=DI_CH00-07  OutputAsBus=on
  Conditioning : Subsystem
  DigitalIn : rtio_opalrt_common/DigitalIn  CtrlName='OpCtrl'  portNb=5  FcnNos=Slot 3 Module A Subsection 1  size=1  maxcount=8  count=8  sampleTime=0  numchan=8
      settings: AttributesFormatString=%<CtrlName>
  DigitalOut : rtio_opalrt_common/DigitalOut  CtrlName='OpCtrl'  portNb=5  FcnNos=Slot 3 Module B Subsection 1  size=1  maxcount=8  count=8  numchan=8
      settings: AttributesFormatString=%<CtrlName>
  Terminator3 : Terminator
  Terminator5 : Terminator
  DIn : Outport
  wires:
  Conditioning/1(Out1) -> Bus Creator/1
  Bus Creator/1 -> DIn/1
  DigitalIn/1 -> Conditioning/1(In1)  "DI_CH00-07"
  DigitalIn/2 -> Terminator5/1
  Bus Selector/1 -> DigitalOut/1
  Dout/1 -> Bus Selector/1
  DigitalOut/1 -> Terminator3/1

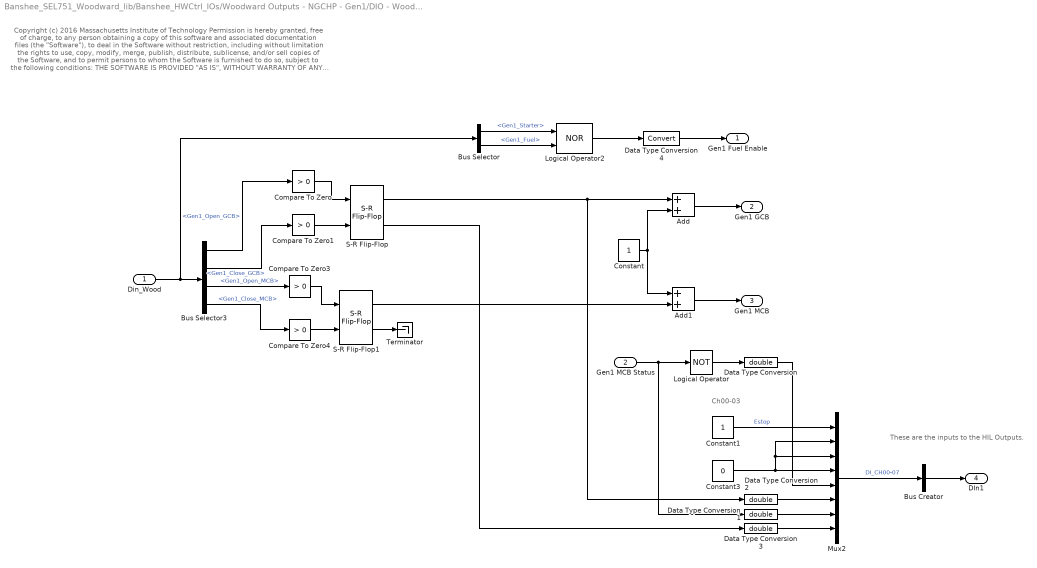
== system Banshee_SEL751_Woodward_lib/Banshee_HWCtrl_IOs/Woodward Outputs - NGCHP - Gen1/DIO - Woodward ==
  note: Copyright (c) 2016 Massachusetts Institute of Technology
      | Permission is hereby granted, free of charge, to any person obtaining a copy of this software and associated documentation files (the "Software"), to deal
      | in the Software without restriction, including without limitation the rights to use, copy, modify, merge, publish, distribute, sublicense, and/or sell copies of the
      | Software, and to permit persons to whom the Software is furnished to do so, subject to the following conditions:
      |
      | THE SOFTWARE IS PROVIDED "AS IS", WITHOUT WARRANTY OF ANY KIND, EXPRESS OR IMPLIED, INCLUDING BUT NOT LIMITED TO THE
      | WARRANTIES OF MERCHANTABILITY, FITNESS FOR A PARTICULAR PURPOSE AND NONINFRINGEMENT. IN NO EVENT SHALL THE AUTHORS
      | OR COPYRIGHT HOLDERS BE LIABLE FOR ANY CLAIM, DAMAGES OR OTHER LIABILITY, WHETHER IN AN ACTION OF CONTRACT, TORT OR
      | OTHERWISE, ARISING FROM, OUT OF OR IN CONNECTION WITH THE SOFTWARE OR THE USE OR OTHER DEALINGS IN THE SOFTWARE
  note: Ch00-03
  note: These are the inputs to
      | the HIL Outputs.
  Din_Wood : Inport
  Gen1 MCB Status : Inport  Port=2
  Add : Sum
  Add1 : Sum
  Bus Creator : BusCreator  Inputs=1
  Bus Selector : BusSelector  OutputSignals=DI_CH00-07.Gen1_Starter,DI_CH00-07.Gen1_Fuel
  Bus Selector3 : BusSelector  OutputSignals=DI_CH00-07.Gen1_Open_GCB,DI_CH00-07.Gen1_Close_GCB,DI_CH00-07.Gen1_Open_MCB,DI_CH00-07.Gen1_Close_MCB
  Compare To Zero{,1,3..4} (4 alike) : simulink/Logic and Bit Operations/Compare To Zero  relop=>  OutDataTypeStr=boolean
  Constant : Constant
  Constant1 : Constant
  Constant3 : Constant  Value=0
  Data Type Conversion{,1..3} (4 alike) : DataTypeConversion  OutDataTypeStr=double
  Data Type Conversion4 : DataTypeConversion
  Logical Operator : Logic  Operator=NOT  AllPortsSameDT=off  OutDataTypeStr=boolean
  Logical Operator2 : Logic  Operator=NOR  AllPortsSameDT=off  OutDataTypeStr=boolean
  Mux2 : Mux  Inputs=8
  S-R Flip-Flop : simulink_extras/Flip Flops/S-R Flip-Flop  initial_condition=1
  S-R Flip-Flop1 : simulink_extras/Flip Flops/S-R Flip-Flop  initial_condition=1
  Terminator : Terminator
  Gen1 Fuel Enable : Outport
  Gen1 GCB : Outport  Port=2
  Gen1 MCB : Outport  Port=3
  DIn1 : Outport  Port=4
  wires:
  S-R Flip-Flop1/2 -> Terminator/1
  Data Type Conversion2/1 -> Mux2/6
  Data Type Conversion1/1 -> Mux2/7
  Data Type Conversion3/1 -> Mux2/8
  Mux2/1 -> Bus Creator/1  "DI_CH00-07"
  Constant3/1 -> Mux2/2, Mux2/3, Mux2/4
  Logical Operator2/1 -> Data Type Conversion4/1
  Logical Operator/1 -> Data Type Conversion/1
  Data Type Conversion/1 -> Mux2/5
  S-R Flip-Flop/2 -> Data Type Conversion3/1
  Gen1 MCB Status/1 -> Logical Operator/1, Data Type Conversion1/1
  Bus Selector3/3 -> Compare To Zero3/1  "<Gen1_Open_MCB>"
  Bus Selector/2 -> Logical Operator2/2  "<Gen1_Fuel>"
  Bus Selector/1 -> Logical Operator2/1  "<Gen1_Starter>"
  Constant/1 -> Add1/1, Add/2
  Add1/1 -> Gen1 MCB/1
  Add/1 -> Gen1 GCB/1
  S-R Flip-Flop1/1 -> Add1/2
  Compare To Zero3/1 -> S-R Flip-Flop1/1
  Compare To Zero4/1 -> S-R Flip-Flop1/2
  Bus Selector3/4 -> Compare To Zero4/1  "<Gen1_Close_MCB>"
  Compare To Zero1/1 -> S-R Flip-Flop/2
  Compare To Zero/1 -> S-R Flip-Flop/1
  S-R Flip-Flop/1 -> Data Type Conversion2/1, Add/1
  Bus Creator/1 -> DIn1/1
  Din_Wood/1 -> Bus Selector/1, Bus Selector3/1
  Bus Selector3/1 -> Compare To Zero/1  "<Gen1_Open_GCB>"
  Bus Selector3/2 -> Compare To Zero1/1  "<Gen1_Close_GCB>"
  Data Type Conversion4/1 -> Gen1 Fuel Enable/1
  Constant1/1 -> Mux2/1  "Estop"

== system Banshee_SEL751_Woodward_lib/Banshee_HWCtrl_IOs/Woodward Outputs - NGCHP - Gen1/DOUT type config ==
  note: The Constants are used to select Digital Output type:
      | - 0: Time-Stamped Digital Output
      | - 1: Pulse-Width Modulated DIgital Output
  DataIn Send : rtio_opalrt_common/DataIn Send  CtrlName='OpCtrl'  FcnNos=11  width=1  portType=double  checkVersion=off  expectedId=0  expectedVersion=0  opComp=>=
      settings: AttributesFormatString=%<CtrlName>
  Subsection 3 DOUT type : Constant
  Terminator2 : Terminator
  wires:
  DataIn Send/1 -> Terminator2/1
  Subsection 3 DOUT type/1 -> DataIn Send/1
